simulink model "constantSetpoints_th"  (R2018b)
settings: Solver=VariableStepAuto  StartTime=0.0  StopTime=10.0  RelTol=1e-3
values from neighbouring files (symbols this model uses):
  CoMPositionVec_cm = [0 0 39]    [constantSetpoints_ts.m]
  faultStatus = false    [constantSetpoints_ts.m]
  pitch_deg = 0    [constantSetpoints_ts.m]
  roll_deg = 1    [constantSetpoints_ts.m]
  yaw_deg = 0    [constantSetpoints_ts.m]
libraries: constantSetpoints_cl x1
settings Model: Creator=mcobb  LastModifiedBy=mcobb

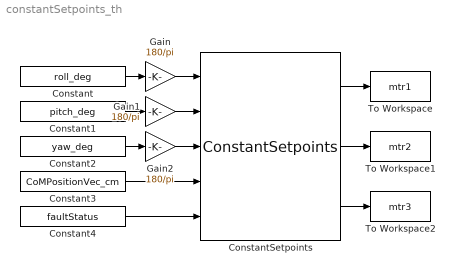
== system constantSetpoints_th ==
  Constant : Constant  Value=roll_deg
  Constant1 : Constant  Value=pitch_deg
  Constant2 : Constant  Value=yaw_deg
  Constant3 : Constant  Value=CoMPositionVec_cm
  Constant4 : Constant  Value=faultStatus
  ConstantSetpoints : constantSetpoints_cl/ConstantSetpoints  SystemSampleTime=-1
  Gain : Gain  Gain=180/pi
  Gain1 : Gain  Gain=180/pi
  Gain2 : Gain  Gain=180/pi
  To Workspace : ToWorkspace  VariableName=mtr1  SaveFormat=Timeseries  SampleTime=-1
  To Workspace1 : ToWorkspace  VariableName=mtr2  SaveFormat=Timeseries  SampleTime=-1
  To Workspace2 : ToWorkspace  VariableName=mtr3  SaveFormat=Timeseries  SampleTime=-1
  wires:
  Constant/1 -> Gain/1
  Constant1/1 -> Gain1/1
  Constant2/1 -> Gain2/1
  Constant3/1 -> ConstantSetpoints/4
  Constant4/1 -> ConstantSetpoints/5
  ConstantSetpoints/1 -> To Workspace/1
  ConstantSetpoints/2 -> To Workspace1/1
  ConstantSetpoints/3 -> To Workspace2/1
  Gain/1 -> ConstantSetpoints/1
  Gain1/1 -> ConstantSetpoints/2
  Gain2/1 -> ConstantSetpoints/3
